simulink model "wireless"  (R2022b)
settings: Solver=ode45  StartTime=0.0  StopTime=50  RelTol=1e-3  EnableMultiTasking=on
InitFcn:
  | clear functions
undefined symbols (not defined in the file or in its folder): ZigBee
libraries: truetime x3, simulink x1
settings Model: Creator=anton  LastModifiedBy=12524
settings SolverCC: AlgebraicLoopSolver=TrustRegion
settings DataIOCC: LimitDataPoints=on  SaveFormat=Array  SignalLoggingSaveFormat=ModelDataLogs  SaveOutput=off  SaveTime=off  ReturnWorkspaceOutputs=off
settings OptimizationCC: BlockReduction=off  BooleanDataType=off  ExpressionDepthLimit=2147483647  LifeSpan=inf
settings DebuggingCC: SaveWithParameterizedLinksMsg=none  UnderspecifiedInitializationDetection=Classic  MergeDetectMultiDrivingBlocksExec=none  SignalResolutionControl=TryResolveAllWithWarning  MultiTaskDSMMsg=warning  MultiTaskCondExecSysMsg=none  FcnCallInpInsideContextMsg=warning  UnconnectedInputMsg=warning  UnconnectedOutputMsg=warning  UnconnectedLineMsg=warning  StateNameClashWarn=warning  SFUnexpectedBacktrackingDiag=warning  SFNoUnconditionalDefaultTransitionDiag=warning  SFExecutionAtInitializationDiag=none  SFMachineParentedDataDiag=warning  ArithmeticOperatorsInVariantConditions=warning
settings HardwareCC: ProdBitPerPointer=32  ProdBitPerSizeT=32  ProdBitPerPtrDiffT=32  ProdLargestAtomicFloat=None  ProdIntDivRoundTo=Undefined  ProdEndianess=Unspecified  ProdWordSize=32  ProdHWDeviceType=32-bit Generic  TargetUnknown=on
settings ModelReferenceCC: PropagateSignalLabelsOutOfModel=off
settings SFSimCC: SimUseLocalCustomCode=off  CustomCodeUndefinedFunction=UseInterfaceOnly
settings RTWCC: RTWUseLocalCustomCode=off
settings CodeAppCC: StateflowObjectComments=on
settings GRTTargetCC: TargetFcnLib=ansi_tfl_tmw.mat  TargetLangStandard=C89/C90 (ANSI)  CombineOutputUpdateFcns=off  GRTInterface=on
settings ConfigComp: CovMetricSettings=dw  CovSaveCumulativeToWorkspaceVar=on  CovSaveSingleToWorkspaceVar=on  CovExternalEMLEnable=off

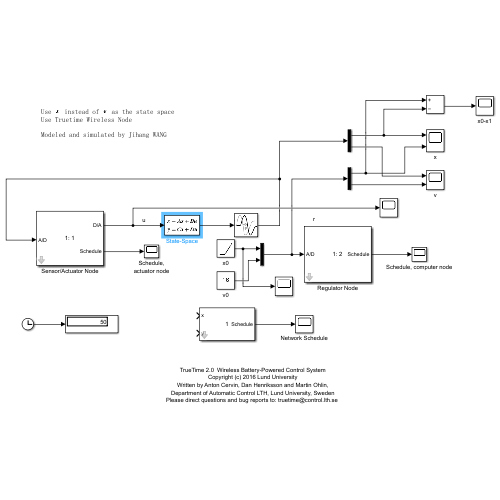
[thumbnail: Simulink's stored preview of the top-level diagram]
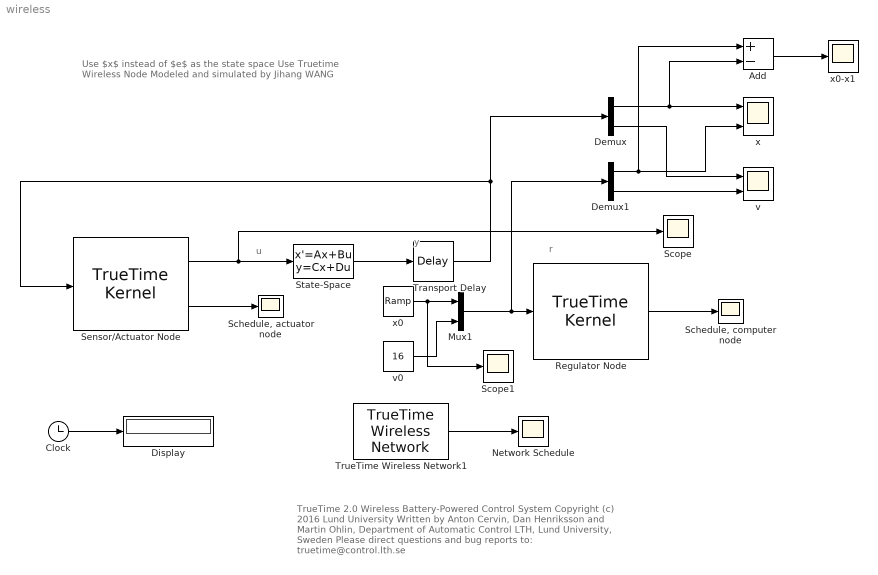
== system wireless ==
  note: Use $x$ instead of $e$ as the state space
      | Use Truetime Wireless Node
      |
      | Modeled and simulated by Jihang WANG
  note: u
  note: y
  note: r
  note: TrueTime 2.0  Wireless Battery-Powered Control System
      | Copyright (c) 2016 Lund University
      | Written by Anton Cervin, Dan Henriksson and Martin Ohlin,
      | Department of Automatic Control LTH, Lund University, Sweden
      | Please direct questions and bug reports to: truetime@control.lth.se
  Add : Sum  Inputs=+-
  Clock : Clock
  Demux : Demux  Outputs=2
  Demux1 : Demux  Outputs=2
  Display : Display
  Mux1 : Mux  Inputs=2
  Network Schedule : Scope
  Regulator Node : truetime/TrueTime Kernel  sfun=regulator_init  args=[]  ninputsoutputs=[2 0]  ntriggers=0  trigtype=falling  nwnodenbr=2  clockoffsetdrift=[0 0]  schedoutput=on  battery=off  poweroutput=off  label=1: 2
  "Schedule, actuator node" : Scope
  "Schedule, computer node" : Scope
  Scope : Scope
  Scope1 : Scope
  Sensor/Actuator Node : truetime/TrueTime Kernel  sfun=actuator_init  args=[]  ninputsoutputs=[2 1]  ntriggers=0  trigtype=falling  nwnodenbr=1  clockoffsetdrift=[0 0]  schedoutput=on  battery=off  poweroutput=off  label=1: 1
  State-Space : StateSpace  A="[0 1 0; 0  0 1; 0 0 -4]"  B=[0; 0; -4]  C=[1 0 0; 0 1 0]  D=[0; 0]  InitialCondition=[-20; 10; 0]
  Transport Delay : TransportDelay  DelayTime=0
  TrueTime Wireless Network1 : truetime/TrueTime Wireless  Network  nwtype=802.15.4 (ZigBee)  nwnbr=1  nnodes=2  rate=800000  minsize=272  transpower=30  threshold=-48  use_pathloss_function=default  pathloss=3.5  acktimeout=0.00004  retrylimit=5  error_threshold=0.03  lossprob=0.6  seed=0  scheduleoutput=on  poweroutput=off
  v : Scope  NumInputPorts=2
  v0 : Constant  Value=16
  x : Scope  NumInputPorts=2
  x0 : simulink/Sources/Ramp  slope=16  start=0  InitialOutput=-10
  x0-x1 : Scope
  wires:
  Clock/1 -> Display/1
  State-Space/1 -> Transport Delay/1
  Sensor/Actuator Node/2 -> "Schedule, actuator node"/1
  Regulator Node/1 -> "Schedule, computer node"/1
  Sensor/Actuator Node/1 -> State-Space/1, Scope/1
  TrueTime Wireless Network1/1 -> Network Schedule/1
  Transport Delay/1 -> Demux/1, Sensor/Actuator Node/1
  x0/1 -> Scope1/1, Mux1/1
  v0/1 -> Mux1/2
  Mux1/1 -> Demux1/1, Regulator Node/1
  Demux/1 -> Add/2, x/1
  Demux1/1 -> Add/1, x/2
  Demux1/2 -> v/2
  Demux/2 -> v/1
  Add/1 -> x0-x1/1
